simulink model "VSI"  (Simulink 7.6)
settings: Solver=ode23tb  StartTime=0  StopTime=10  MaxStep=5e-6  RelTol=1e-4  AbsTol=1e-5
InitFcn:
  | clear all
  | VSI_AFE_parameters_G1_s
values from neighbouring files (symbols this model uses):
  Cdc_afe = 98.8e-6    (= 9.88e-05)    [VSI_AFE_parameters_G1_s.m]
  DeadTime = 0.0e-6    (= 0)    [VSI_AFE_parameters_G1_s.m]
  f = 400    [VSI_AFE_parameters_G1_s.m]
  La = 1000e-6    (= 0.001)    [VSI_AFE_parameters_G1_s.m]
  Lb = 1000e-6    (= 0.001)    [VSI_AFE_parameters_G1_s.m]
  Lboost_a = 474e-6    (= 0.000474)    [VSI_AFE_parameters_G1_s.m]
  Lboost_b = 471e-6    (= 0.000471)    [VSI_AFE_parameters_G1_s.m]
  Lboost_c = 463e-6    (= 0.000463)    [VSI_AFE_parameters_G1_s.m]
  Lc = 1000e-6    (= 0.001)    [VSI_AFE_parameters_G1_s.m]
  LCdc_afe = 0.65e-6    (= 6.5e-07)    [VSI_AFE_parameters_G1_s.m]
  PWM_Cycle = 4000    [VSI_AFE_parameters_G1_s.m]
  RCdc_afe = 0.049    [VSI_AFE_parameters_G1_s.m]
  Rdc = 96    [VSI_AFE_parameters_G1_s.m]
  RLa = 0.100    (= 0.1)    [VSI_AFE_parameters_G1_s.m]
  RLb = 0.100    (= 0.1)    [VSI_AFE_parameters_G1_s.m]
  RLboost_a = 0.080    (= 0.08)    [VSI_AFE_parameters_G1_s.m]
  RLboost_b = 0.084    [VSI_AFE_parameters_G1_s.m]
  RLboost_c = 0.110    (= 0.11)    [VSI_AFE_parameters_G1_s.m]
  RLc = 0.100    (= 0.1)    [VSI_AFE_parameters_G1_s.m]
  Vdc = 270/1    (= 270)    [VSI_AFE_parameters_G1_s.m]
  Vfd = 0.75    [VSI_AFE_parameters_G1_s.m]
  Vfs = 1.0    (= 1)    [VSI_AFE_parameters_G1_s.m]
  Vsm = Vse*sqrt(2)-8.2/sqrt(2)*Rss    [VSI_AFE_parameters_G1_s.m]
undefined symbols (not defined in the file or in its folder): Cdc, Ldc
libraries: powerlib x55, cstblocks x10, simulink x4, powerlib_extras x1
settings Model: Creator=marko  LastModifiedBy=wenbo
settings SolverCC: MaxConsecutiveMinStep=10  ZeroCrossAlgorithm=Adaptive  AlgebraicLoopSolver=LineSearch
settings DataIOCC: LimitDataPoints=off  SaveOutput=off  SaveTime=off
settings DebuggingCC: IgnoredZcDiagnostic=none  StrictBusMsg=Warning

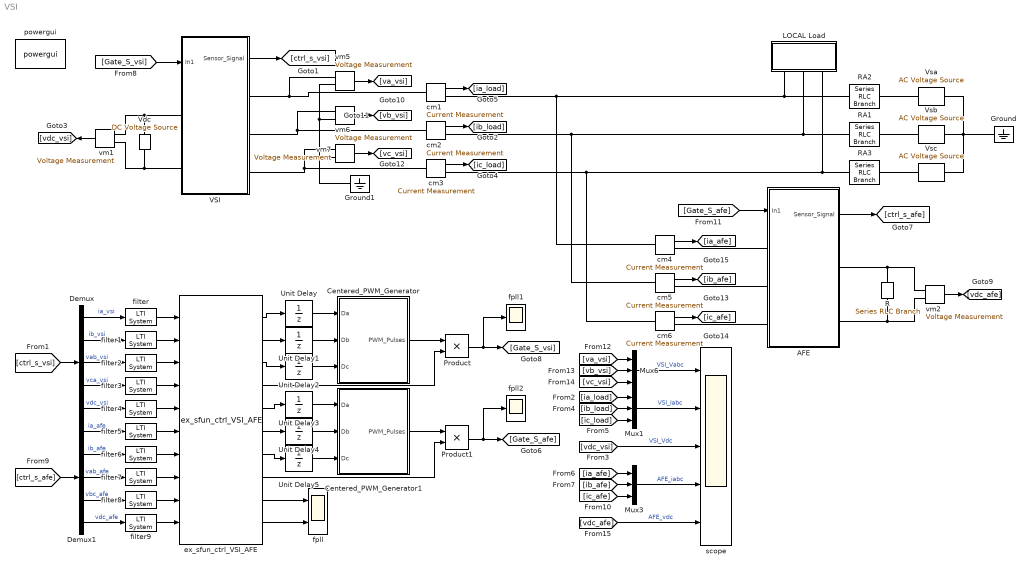
== system VSI ==
  AFE : Subsystem
  Centered_PWM_Generator : Subsystem
  Centered_PWM_Generator1 : Subsystem
  Demux : Demux  Outputs=5
  Demux1 : Demux  Outputs=5
  Ground : powerlib/Elements/Ground  DialogController=POWERSYS.PowerSysDialog  PhysicalDomain=powersysdomain  SubClassName=unknown  LeftPortType=p1  RightPortType=p1  LConnTagsString=a
  Ground1 : powerlib/Elements/Ground  DialogController=POWERSYS.PowerSysDialog  PhysicalDomain=powersysdomain  SubClassName=unknown  LeftPortType=p1  RightPortType=p1  LConnTagsString=a
  LOCAL Load : Subsystem
  Mux1 : Mux  Inputs=3
  Mux3 : Mux  Inputs=3
  Mux6 : Mux  Inputs=3
  Product : Product  RndMeth=Zero
  Product1 : Product  RndMeth=Zero
  R : powerlib/Elements/Series RLC Branch  DialogController=POWERSYS.PowerSysDialog  PhysicalDomain=powersysdomain  SubClassName=unknown  LeftPortType=p1  RightPortType=p1  LConnTagsString=__new0  RConnTagsString=__new0  BranchType=R  Resistance=Rdc  Inductance=Ldc  SetiL0=off  InitialCurrent=0  Capacitance=Cdc  Setx0=off  InitialVoltage=0  Measurements=None
  RA1 : powerlib/Elements/Series RLC Branch  DialogController=POWERSYS.PowerSysDialog  PhysicalDomain=powersysdomain  SubClassName=unknown  LeftPortType=p1  RightPortType=p1  LConnTagsString=__new0  RConnTagsString=__new0  BranchType=R  Resistance=10  Inductance=1e-3  SetiL0=off  InitialCurrent=0  Capacitance=1e-6  Setx0=off  InitialVoltage=0  Measurements=None
  RA2 : powerlib/Elements/Series RLC Branch  DialogController=POWERSYS.PowerSysDialog  PhysicalDomain=powersysdomain  SubClassName=unknown  LeftPortType=p1  RightPortType=p1  LConnTagsString=__new0  RConnTagsString=__new0  BranchType=R  Resistance=10  Inductance=1e-3  SetiL0=off  InitialCurrent=0  Capacitance=1e-6  Setx0=off  InitialVoltage=0  Measurements=None
  RA3 : powerlib/Elements/Series RLC Branch  DialogController=POWERSYS.PowerSysDialog  PhysicalDomain=powersysdomain  SubClassName=unknown  LeftPortType=p1  RightPortType=p1  LConnTagsString=__new0  RConnTagsString=__new0  BranchType=R  Resistance=10  Inductance=1e-3  SetiL0=off  InitialCurrent=0  Capacitance=1e-6  Setx0=off  InitialVoltage=0  Measurements=None
  Unit Delay{,1..5} (6 alike) : UnitDelay  SampleTime=-1
  VSI : Subsystem
  Vdc : powerlib/Electrical Sources/DC Voltage Source  DialogController=POWERSYS.PowerSysDialog  SystemSampleTime=-1  Amplitude=Vdc  Measurements=None
  Vsa : powerlib/Electrical Sources/AC Voltage Source  DialogController=POWERSYS.PowerSysDialog  SystemSampleTime=-1  Amplitude=Vsm  Phase=90  Frequency=f  SampleTime=0  Measurements=None
  Vsb : powerlib/Electrical Sources/AC Voltage Source  DialogController=POWERSYS.PowerSysDialog  SystemSampleTime=-1  Amplitude=Vsm  Phase=90-120  Frequency=f  SampleTime=0  Measurements=None
  Vsc : powerlib/Electrical Sources/AC Voltage Source  DialogController=POWERSYS.PowerSysDialog  SystemSampleTime=-1  Amplitude=Vsm  Phase=90+120  Frequency=f  SampleTime=0  Measurements=None
  cm{1..6} (6 alike) : powerlib/Measurements/Current Measurement  DialogController=POWERSYS.PowerSysDialog  SystemSampleTime=-1  PhasorSimulation=off  OutputType=Complex  PSBequivalent=0
  ex_sfun_ctrl_VSI_AFE : S-Function  FunctionName=ex_sfun_ctrl_VSI_AFE  EnableBusSupport=off  mask(Legacy Function){SFunctionSpec=void epwm1_isr(double y1[1], double y2[1], double y3[1], double y4[1], double y5[1], double y6[1], double y7[1], double y8[1], double y9[1], double u1, double u2, double u3, double u4, double u5, double u6, double u7, double u8, double u9, double u10), ShowSpec=off}
      mask prompts: ShowSpec "Display function specification"
      mask help:
      | This block allows you to call the legacy functions specified by the following Legacy Code Tool definition:
      | def.SFunctionName = 'ex_sfun_ctrl_VSI_AFE';
      | def.OutputFcnSpec = 'void epwm1_isr(double y1[1], double y2[1], double y3[1], double y4[1], double y5[1], double y6[1], double y7[1], double y8[1], double y9[1], double u1, double u2, double u3, double u4, double u5, double u6, double u7, double u8, double u9, double u10)';
      | def.HeaderFiles = {'math.h'};
      | def.SourceFiles = {'epwm1_isr.c'};
      | def.SampleTime = 5e-005;
      mask Help: <p>This block was generated automatically by the Legacy Code Tool. For detailed help on this tool, call<a href="matlab:legacy_code('help')"> legacy_code('help')</a>.</p>
      mask CallbackString:
      | |if strcmp(get_param(gcbh, 'ShowSpec'), 'on')
      |   set_param(gcbh, 'MaskDisplay', sprintf('fprintf(''%s'');', get_param(gcbh, 'SFunctionSpec')));
      | else
      |   set_param(gcbh, 'MaskDisplay', sprintf('fprintf(''%s'');', get_param(gcbh, 'FunctionName')));
      | end
      mask Display: fprintf('ex_sfun_ctrl_VSI_AFE');
  filter{,1..9} (10 alike) : cstblocks/LTI System  SystemSampleTime=-1  sys=tf_filter  IC=[]
  fpll : Scope  NumInputPorts=2
      settings: TimeRange=10  YMin=375~373  YMax=378.25~379.5  SaveName=ia_L
  fpll1 : Scope
      settings: TimeRange=1  YMin=358.141  YMax=395.841  SaveName=ia_L1
  fpll2 : Scope
      settings: TimeRange=1  YMin=358.141  YMax=395.841  SaveName=ia_L2
  powergui : powerlib/powergui  Priority=1  SystemSampleTime=-1  SimulationMode=Continuous  SampleTime=50e-6  frequency=60  SPID=on  DisableSnubberDevices=off  DisableRonSwitches=off  DisableVfSwitches=off  SwTol=0  Interpol=off  frequencyindice=0  echomessages=off  HookPort=off  DisplayEquations=off  FunctionMessages=off  EnableUseOfTLC=off  x0status=blocks  RestoreLinks=warning  ResistiveCurrentMeasurement=off  Frange=[0:2:500]  Ylog=off  Xlog=on  ShowGrid=off  save=off  variable=ZData  structure=ia_L  ZoomFFT=on  StartTime=0.1  cycles=1  DisplayStyle=1  fundamental=400  FreqAxis=off  MaxFrequency=100000  frequencyindicesteady=400  RmsSteady=1  display=off  Ts=0  methode=off
  scope : Scope  NumInputPorts=5
      settings: TimeRange=10  YMin=-100~-15~256.5~-15~0  YMax=100~17.5~283.5~25~250  SaveName=va_ia  MaxDataPoints=2000000
  vm{1..2,5..7} (5 alike) : powerlib/Measurements/Voltage Measurement  DialogController=POWERSYS.PowerSysDialog  SystemSampleTime=-1  PhasorSimulation=off  OutputType=Complex  PSBequivalent=0
  wires:
  vm5/1 -> [va_vsi]
  vm6/1 -> [vb_vsi]
  vm7/1 -> [vc_vsi]
  [va_vsi] -> Mux6/1
  [vb_vsi] -> Mux6/2
  [vc_vsi] -> Mux6/3
  Mux6/1 -> scope/1  "VSI_Vabc"
  Unit Delay/1 -> Centered_PWM_Generator/1(Da)
  Unit Delay1/1 -> Centered_PWM_Generator/2(Db)
  Unit Delay2/1 -> Centered_PWM_Generator/3(Dc)
  Demux/1 -> filter/1  "ia_vsi"
  Demux/2 -> filter1/1  "ib_vsi"
  Demux/3 -> filter2/1  "vab_vsi"
  Demux/4 -> filter3/1  "vca_vsi"
  Demux/5 -> filter4/1  "vdc_vsi"
  VSI/1(Sensor_Signal) -> [ctrl_s_vsi]
  [ctrl_s_vsi] -> Demux/1
  [Gate_S_vsi] -> VSI/1(In1)
  Demux1/1 -> filter5/1  "ia_afe"
  Demux1/2 -> filter6/1  "ib_afe"
  Demux1/3 -> filter7/1  "vab_afe"
  Demux1/4 -> filter8/1  "vbc_afe"
  Demux1/5 -> filter9/1  "vdc_afe"
  [ctrl_s_afe] -> Demux1/1
  ex_sfun_ctrl_VSI_AFE/1 -> Unit Delay/1
  ex_sfun_ctrl_VSI_AFE/2 -> Unit Delay1/1
  ex_sfun_ctrl_VSI_AFE/3 -> Unit Delay2/1
  filter/1 -> ex_sfun_ctrl_VSI_AFE/1
  filter1/1 -> ex_sfun_ctrl_VSI_AFE/2
  filter2/1 -> ex_sfun_ctrl_VSI_AFE/3
  filter3/1 -> ex_sfun_ctrl_VSI_AFE/4
  filter4/1 -> ex_sfun_ctrl_VSI_AFE/5
  filter5/1 -> ex_sfun_ctrl_VSI_AFE/6
  filter6/1 -> ex_sfun_ctrl_VSI_AFE/7
  filter7/1 -> ex_sfun_ctrl_VSI_AFE/8
  filter8/1 -> ex_sfun_ctrl_VSI_AFE/9
  filter9/1 -> ex_sfun_ctrl_VSI_AFE/10
  cm1/1 -> [ia_load]
  [vdc_vsi] -> scope/3  "VSI_Vdc"
  vm1/1 -> [vdc_vsi]
  cm2/1 -> [ib_load]
  cm3/1 -> [ic_load]
  Mux1/1 -> scope/2  "VSI_Iabc"
  [ia_load] -> Mux1/1
  [ib_load] -> Mux1/2
  [ic_load] -> Mux1/3
  Product/1 -> [Gate_S_vsi], fpll1/1
  Centered_PWM_Generator/1(PWM_Pulses) -> Product/1
  ex_sfun_ctrl_VSI_AFE/9 -> fpll/1
  ex_sfun_ctrl_VSI_AFE/10 -> fpll/2
  ex_sfun_ctrl_VSI_AFE/4 -> Product/2
  Unit Delay3/1 -> Centered_PWM_Generator1/1(Da)
  Unit Delay4/1 -> Centered_PWM_Generator1/2(Db)
  Unit Delay5/1 -> Centered_PWM_Generator1/3(Dc)
  Product1/1 -> fpll2/1, [Gate_S_afe]
  Centered_PWM_Generator1/1(PWM_Pulses) -> Product1/1
  ex_sfun_ctrl_VSI_AFE/8 -> Product1/2
  ex_sfun_ctrl_VSI_AFE/5 -> Unit Delay3/1
  ex_sfun_ctrl_VSI_AFE/6 -> Unit Delay4/1
  ex_sfun_ctrl_VSI_AFE/7 -> Unit Delay5/1
  [ia_afe] -> Mux3/1
  [ib_afe] -> Mux3/2
  [ic_afe] -> Mux3/3
  Mux3/1 -> scope/4  "AFE_iabc"
  [vdc_afe] -> scope/5  "AFE_vdc"
  [Gate_S_afe] -> AFE/1(In1)
  AFE/1(Sensor_Signal) -> [ctrl_s_afe]
  vm2/1 -> [vdc_afe]
  cm4/1 -> [ia_afe]
  cm5/1 -> [ib_afe]
  cm6/1 -> [ic_afe]
  connections:
  VSI/LConn1 -- Vdc/RConn1 -- vm1/LConn1
  VSI/LConn2 -- Vdc/LConn1 -- vm1/LConn2
  VSI/RConn3 -- vm7/LConn1 -- cm3/LConn1
  VSI/RConn2 -- vm6/LConn1 -- cm2/LConn1
  cm1/LConn1 -- VSI/RConn1 -- vm5/LConn1
  RA2/RConn1 -- LOCAL Load/LConn1 -- cm1/RConn1 -- cm4/LConn1
  RA1/RConn1 -- LOCAL Load/LConn2 -- cm2/RConn1 -- cm5/LConn1
  RA3/RConn1 -- LOCAL Load/LConn3 -- cm3/RConn1 -- cm6/LConn1
  Vsa/LConn1 -- Vsc/LConn1 -- Vsb/LConn1 -- Ground/LConn1
  vm5/LConn2 -- vm6/LConn2 -- Ground1/LConn1 -- vm7/LConn2
  RA2/LConn1 -- Vsa/RConn1
  Vsb/RConn1 -- RA1/LConn1
  Vsc/RConn1 -- RA3/LConn1
  AFE/RConn2 -- R/RConn1 -- vm2/LConn2
  AFE/RConn1 -- R/LConn1 -- vm2/LConn1
  AFE/LConn1 -- cm4/RConn1
  AFE/LConn2 -- cm5/RConn1
  AFE/LConn3 -- cm6/RConn1

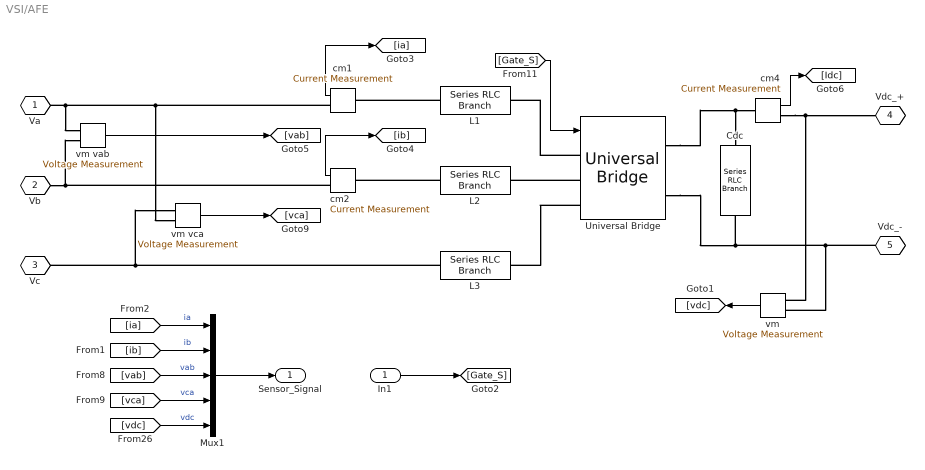
== system VSI/AFE ==
  In1 : Inport
  Cdc : powerlib/Elements/Series RLC Branch  DialogController=POWERSYS.PowerSysDialog  PhysicalDomain=powersysdomain  SubClassName=unknown  LeftPortType=p1  RightPortType=p1  LConnTagsString=__new0  RConnTagsString=__new0  BranchType=C  Resistance=RCdc_afe  Inductance=LCdc_afe  SetiL0=off  InitialCurrent=0  Capacitance=Cdc_afe  Setx0=off  InitialVoltage=0  Measurements=None
  L1 : powerlib/Elements/Series RLC Branch  DialogController=POWERSYS.PowerSysDialog  PhysicalDomain=powersysdomain  SubClassName=unknown  LeftPortType=p1  RightPortType=p1  LConnTagsString=__new0  RConnTagsString=__new0  BranchType=RL  Resistance=RLboost_a  Inductance=Lboost_a  SetiL0=off  InitialCurrent=0  Capacitance=1e-6  Setx0=off  InitialVoltage=0  Measurements=None
  L2 : powerlib/Elements/Series RLC Branch  DialogController=POWERSYS.PowerSysDialog  PhysicalDomain=powersysdomain  SubClassName=unknown  LeftPortType=p1  RightPortType=p1  LConnTagsString=__new0  RConnTagsString=__new0  BranchType=RL  Resistance=RLboost_b  Inductance=Lboost_b  SetiL0=off  InitialCurrent=0  Capacitance=1e-6  Setx0=off  InitialVoltage=0  Measurements=None
  L3 : powerlib/Elements/Series RLC Branch  DialogController=POWERSYS.PowerSysDialog  PhysicalDomain=powersysdomain  SubClassName=unknown  LeftPortType=p1  RightPortType=p1  LConnTagsString=__new0  RConnTagsString=__new0  BranchType=RL  Resistance=RLboost_c  Inductance=Lboost_c  SetiL0=off  InitialCurrent=0  Capacitance=1e-6  Setx0=off  InitialVoltage=0  Measurements=None
  Mux1 : Mux  Inputs=5
  Universal Bridge : powerlib/Power Electronics/Universal Bridge  DialogController=POWERSYS.PowerSysDialog  SystemSampleTime=-1  Arms=3  SnubberResistance=inf  SnubberCapacitance=inf  Device=IGBT / Diodes  Ron=Rsd  Lon=0  ForwardVoltages=[Vfs Vfd]  ForwardVoltage=0  GTOparameters=[ 10e-6 , 20e-6 ]  IGBTparameters=[ 0, 0 ]  Measurements=None  Measurements_2=None  converterType=Rectifier
  cm1 : powerlib/Measurements/Current Measurement  DialogController=POWERSYS.PowerSysDialog  SystemSampleTime=-1  PhasorSimulation=off  OutputType=Complex  PSBequivalent=0
  cm2 : powerlib/Measurements/Current Measurement  DialogController=POWERSYS.PowerSysDialog  SystemSampleTime=-1  PhasorSimulation=off  OutputType=Complex  PSBequivalent=0
  cm4 : powerlib/Measurements/Current Measurement  DialogController=POWERSYS.PowerSysDialog  SystemSampleTime=-1  PhasorSimulation=off  OutputType=Complex  PSBequivalent=0
  vm : powerlib/Measurements/Voltage Measurement  DialogController=POWERSYS.PowerSysDialog  SystemSampleTime=-1  PhasorSimulation=off  OutputType=Complex  PSBequivalent=0
  vm vab : powerlib/Measurements/Voltage Measurement  DialogController=POWERSYS.PowerSysDialog  SystemSampleTime=-1  PhasorSimulation=off  OutputType=Complex  PSBequivalent=0
  vm vca : powerlib/Measurements/Voltage Measurement  DialogController=POWERSYS.PowerSysDialog  SystemSampleTime=-1  PhasorSimulation=off  OutputType=Complex  PSBequivalent=0
  Va : PMIOPort  Tag=PMCPort  Port=1  Side=Left
  Vb : PMIOPort  Tag=PMCPort  Port=2  Side=Left
  Vc : PMIOPort  Tag=PMCPort  Port=3  Side=Left
  Vdc_+ : PMIOPort  Tag=PMCPort  Port=4  Side=Right
  Vdc_- : PMIOPort  Tag=PMCPort  Port=5  Side=Right
  Sensor_Signal : Outport
  wires:
  [Gate_S] -> Universal Bridge/1
  cm4/1 -> [Idc]
  cm1/1 -> [ia]
  cm2/1 -> [ib]
  vm vab/1 -> [vab]
  vm vca/1 -> [vca]
  vm/1 -> [vdc]
  [ia] -> Mux1/1  "ia"
  [ib] -> Mux1/2  "ib"
  [vab] -> Mux1/3  "vab"
  [vca] -> Mux1/4  "vca"
  [vdc] -> Mux1/5  "vdc"
  Mux1/1 -> Sensor_Signal/1
  In1/1 -> [Gate_S]
  connections:
  Universal Bridge/LConn1 -- L1/RConn1
  Universal Bridge/LConn2 -- L2/RConn1
  Universal Bridge/LConn3 -- L3/RConn1
  vm vab/LConn1 -- cm1/RConn1 -- vm vca/LConn2 -- Va/RConn1
  cm2/RConn1 -- Vb/RConn1 -- vm vab/LConn2
  cm4/RConn1 -- Vdc_+/RConn1 -- vm/LConn1
  Vdc_-/RConn1 -- Universal Bridge/RConn2 -- Cdc/RConn1 -- vm/LConn2
  L1/LConn1 -- cm1/LConn1
  L2/LConn1 -- cm2/LConn1
  L3/LConn1 -- Vc/RConn1 -- vm vca/LConn1
  Universal Bridge/RConn1 -- cm4/LConn1 -- Cdc/LConn1

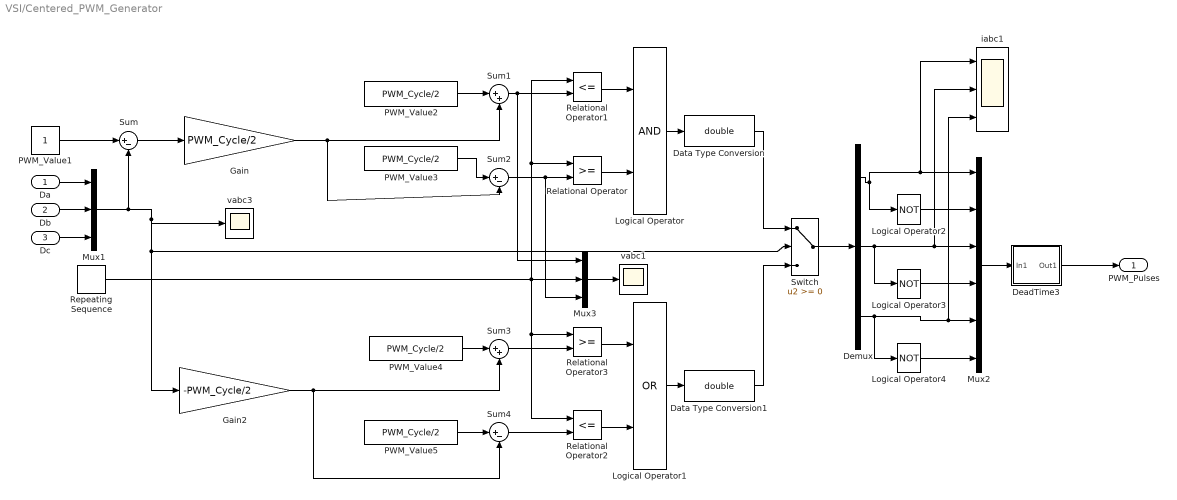
== system VSI/Centered_PWM_Generator ==
  Da : Inport
  Db : Inport  Port=2
  Dc : Inport  Port=3
  Data Type Conversion : DataTypeConversion  OutDataTypeStr=double
  Data Type Conversion1 : DataTypeConversion  OutDataTypeStr=double
  DeadTime3 : Subsystem
  Demux : Demux  Outputs=3
  Gain : Gain  Gain=PWM_Cycle/2
  Gain2 : Gain  Gain=-PWM_Cycle/2
  Logical Operator : Logic  AllPortsSameDT=off  OutDataTypeStr=boolean
  Logical Operator1 : Logic  Operator=OR  AllPortsSameDT=off  OutDataTypeStr=boolean
  Logical Operator2 : Logic  Operator=NOT  OutDataTypeStr=float('double')
  Logical Operator3 : Logic  Operator=NOT  OutDataTypeStr=float('double')
  Logical Operator4 : Logic  Operator=NOT  OutDataTypeStr=float('double')
  Mux1 : Mux  Inputs=3
  Mux2 : Mux  Inputs=6
  Mux3 : Mux  Inputs=3
  PWM_Value1 : Constant
  PWM_Value{2..5} (4 alike) : Constant  Value=PWM_Cycle/2
  Relational Operator : RelationalOperator  OutDataTypeStr=boolean
  Relational Operator1 : RelationalOperator  Operator=<=  OutDataTypeStr=boolean
  Relational Operator2 : RelationalOperator  Operator=<=  OutDataTypeStr=boolean
  Relational Operator3 : RelationalOperator  OutDataTypeStr=boolean
  Repeating Sequence : simulink/Sources/Repeating Sequence  rep_seq_t="[0  (0.5*PWM_Cycle*12.5e-9) (1*PWM_Cycle*12.5e-9)]"  rep_seq_y=[0 PWM_Cycle 0]
  Sum : Sum  Inputs=|+-
  Sum1 : Sum  Inputs=|++
  Sum2 : Sum  Inputs=|+-
  Sum3 : Sum  Inputs=|++
  Sum4 : Sum  Inputs=|+-
  Switch : Switch
  iabc1 : Scope  NumInputPorts=3
      settings: TimeRange=0.02  YMin=-9~-5~-5  YMax=8~5~5  SaveName=iabc_L2
  vabc1 : Scope
      settings: TimeRange=0.01  YMin=0  YMax=4000  SaveName=vabcll2
  vabc3 : Scope
      settings: TimeRange=0.01  YMin=-11  YMax=12  SaveName=vabcll1
  PWM_Pulses : Outport
  wires:
  Logical Operator4/1 -> Mux2/6
  Demux/3 -> Logical Operator4/1, Mux2/5, iabc1/3
  Logical Operator3/1 -> Mux2/4
  Demux/2 -> Logical Operator3/1, Mux2/3, iabc1/2
  Logical Operator2/1 -> Mux2/2
  Demux/1 -> Logical Operator2/1, Mux2/1, iabc1/1
  Mux2/1 -> DeadTime3/1(In1)
  Dc/1 -> Mux1/3
  Db/1 -> Mux1/2
  Da/1 -> Mux1/1
  Mux1/1 -> Sum/2, Switch/2, Gain2/1, vabc3/1
  Switch/1 -> Demux/1
  Data Type Conversion1/1 -> Switch/3
  Gain2/1 -> Sum3/2, Sum4/2
  Logical Operator1/1 -> Data Type Conversion1/1
  Relational Operator2/1 -> Logical Operator1/2
  Relational Operator3/1 -> Logical Operator1/1
  Sum3/1 -> Relational Operator3/2
  Sum4/1 -> Relational Operator2/2
  PWM_Value5/1 -> Sum4/1
  PWM_Value4/1 -> Sum3/1
  Data Type Conversion/1 -> Switch/1
  Logical Operator/1 -> Data Type Conversion/1
  Relational Operator/1 -> Logical Operator/2
  Relational Operator1/1 -> Logical Operator/1
  Sum1/1 -> Relational Operator1/2, Mux3/1
  Sum2/1 -> Relational Operator/2, Mux3/3
  PWM_Value3/1 -> Sum2/1
  Gain/1 -> Sum2/2, Sum1/2
  Sum/1 -> Gain/1
  PWM_Value1/1 -> Sum/1
  Repeating Sequence/1 -> Relational Operator1/1, Relational Operator/1, Relational Operator3/1, Relational Operator2/1, Mux3/2
  DeadTime3/1(Out1) -> PWM_Pulses/1
  PWM_Value2/1 -> Sum1/1
  Mux3/1 -> vabc1/1

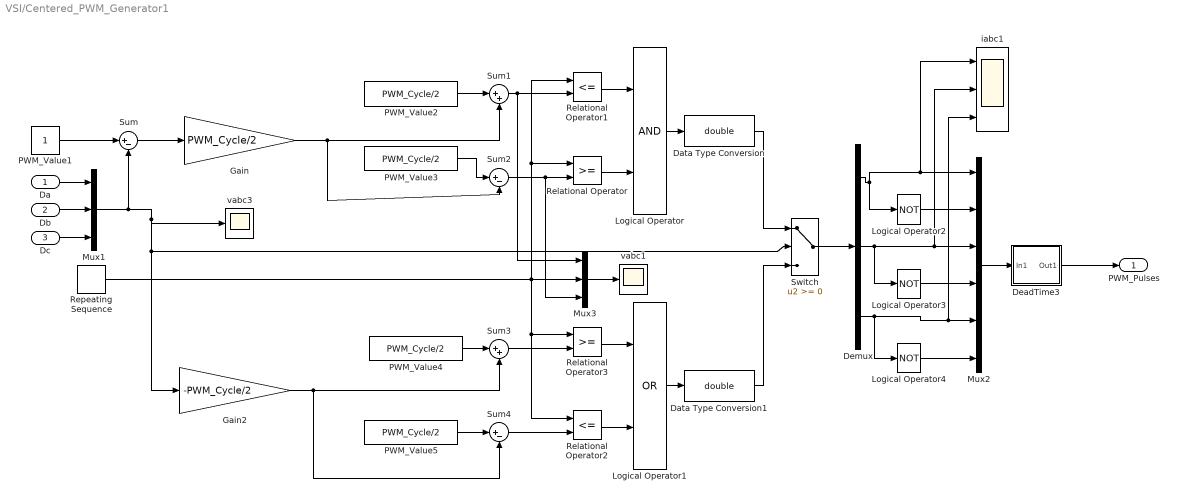
== system VSI/Centered_PWM_Generator1 ==
  Da : Inport
  Db : Inport  Port=2
  Dc : Inport  Port=3
  Data Type Conversion : DataTypeConversion  OutDataTypeStr=double
  Data Type Conversion1 : DataTypeConversion  OutDataTypeStr=double
  DeadTime3 : Subsystem
  Demux : Demux  Outputs=3
  Gain : Gain  Gain=PWM_Cycle/2
  Gain2 : Gain  Gain=-PWM_Cycle/2
  Logical Operator : Logic  AllPortsSameDT=off  OutDataTypeStr=boolean
  Logical Operator1 : Logic  Operator=OR  AllPortsSameDT=off  OutDataTypeStr=boolean
  Logical Operator2 : Logic  Operator=NOT  OutDataTypeStr=float('double')
  Logical Operator3 : Logic  Operator=NOT  OutDataTypeStr=float('double')
  Logical Operator4 : Logic  Operator=NOT  OutDataTypeStr=float('double')
  Mux1 : Mux  Inputs=3
  Mux2 : Mux  Inputs=6
  Mux3 : Mux  Inputs=3
  PWM_Value1 : Constant
  PWM_Value{2..5} (4 alike) : Constant  Value=PWM_Cycle/2
  Relational Operator : RelationalOperator  OutDataTypeStr=boolean
  Relational Operator1 : RelationalOperator  Operator=<=  OutDataTypeStr=boolean
  Relational Operator2 : RelationalOperator  Operator=<=  OutDataTypeStr=boolean
  Relational Operator3 : RelationalOperator  OutDataTypeStr=boolean
  Repeating Sequence : simulink/Sources/Repeating Sequence  rep_seq_t="[0  (0.5*PWM_Cycle*12.5e-9) (1*PWM_Cycle*12.5e-9)]"  rep_seq_y=[0 PWM_Cycle 0]
  Sum : Sum  Inputs=|+-
  Sum1 : Sum  Inputs=|++
  Sum2 : Sum  Inputs=|+-
  Sum3 : Sum  Inputs=|++
  Sum4 : Sum  Inputs=|+-
  Switch : Switch
  iabc1 : Scope  NumInputPorts=3
      settings: TimeRange=0.02  YMin=-9~-5~-5  YMax=8~5~5  SaveName=iabc_L2
  vabc1 : Scope
      settings: TimeRange=0.01  YMin=0  YMax=4000  SaveName=vabcll2
  vabc3 : Scope
      settings: TimeRange=0.01  YMin=-11  YMax=12  SaveName=vabcll1
  PWM_Pulses : Outport
  wires:
  Mux3/1 -> vabc1/1
  PWM_Value2/1 -> Sum1/1
  DeadTime3/1(Out1) -> PWM_Pulses/1
  Repeating Sequence/1 -> Mux3/2, Relational Operator2/1, Relational Operator3/1, Relational Operator/1, Relational Operator1/1
  PWM_Value1/1 -> Sum/1
  Sum/1 -> Gain/1
  Gain/1 -> Sum1/2, Sum2/2
  PWM_Value3/1 -> Sum2/1
  Sum2/1 -> Mux3/3, Relational Operator/2
  Sum1/1 -> Mux3/1, Relational Operator1/2
  Relational Operator1/1 -> Logical Operator/1
  Relational Operator/1 -> Logical Operator/2
  Logical Operator/1 -> Data Type Conversion/1
  Data Type Conversion/1 -> Switch/1
  PWM_Value4/1 -> Sum3/1
  PWM_Value5/1 -> Sum4/1
  Sum4/1 -> Relational Operator2/2
  Sum3/1 -> Relational Operator3/2
  Relational Operator3/1 -> Logical Operator1/1
  Relational Operator2/1 -> Logical Operator1/2
  Logical Operator1/1 -> Data Type Conversion1/1
  Gain2/1 -> Sum4/2, Sum3/2
  Data Type Conversion1/1 -> Switch/3
  Switch/1 -> Demux/1
  Mux1/1 -> vabc3/1, Gain2/1, Switch/2, Sum/2
  Da/1 -> Mux1/1
  Db/1 -> Mux1/2
  Dc/1 -> Mux1/3
  Mux2/1 -> DeadTime3/1(In1)
  Demux/1 -> iabc1/1, Mux2/1, Logical Operator2/1
  Logical Operator2/1 -> Mux2/2
  Demux/2 -> iabc1/2, Mux2/3, Logical Operator3/1
  Logical Operator3/1 -> Mux2/4
  Demux/3 -> iabc1/3, Mux2/5, Logical Operator4/1
  Logical Operator4/1 -> Mux2/6

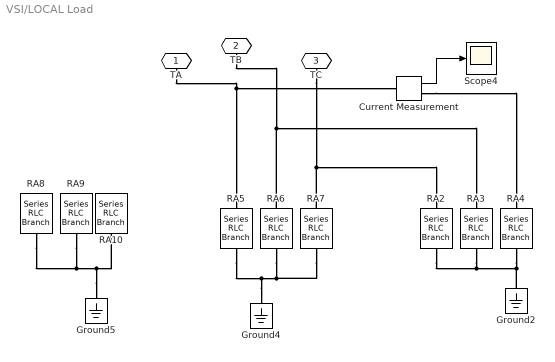
== system VSI/LOCAL Load ==
  Current Measurement : powerlib/Measurements/Current Measurement  DialogController=POWERSYS.PowerSysDialog  SystemSampleTime=-1  PhasorSimulation=off  OutputType=Complex  PSBequivalent=0
  Ground2 : powerlib/Elements/Ground  DialogController=POWERSYS.PowerSysDialog  PhysicalDomain=powersysdomain  SubClassName=unknown  LeftPortType=p1  RightPortType=p1  LConnTagsString=a
  Ground4 : powerlib/Elements/Ground  DialogController=POWERSYS.PowerSysDialog  PhysicalDomain=powersysdomain  SubClassName=unknown  LeftPortType=p1  RightPortType=p1  LConnTagsString=a
  Ground5 : powerlib/Elements/Ground  DialogController=POWERSYS.PowerSysDialog  PhysicalDomain=powersysdomain  SubClassName=unknown  LeftPortType=p1  RightPortType=p1  LConnTagsString=a
  RA10 : powerlib/Elements/Series RLC Branch  DialogController=POWERSYS.PowerSysDialog  PhysicalDomain=powersysdomain  SubClassName=unknown  LeftPortType=p1  RightPortType=p1  LConnTagsString=__new0  RConnTagsString=__new0  BranchType=L  Resistance=0.01e-3  Inductance=80e-3  SetiL0=off  InitialCurrent=0  Capacitance=10e-6  Setx0=off  InitialVoltage=0  Measurements=None
  RA2 : powerlib/Elements/Series RLC Branch  DialogController=POWERSYS.PowerSysDialog  PhysicalDomain=powersysdomain  SubClassName=unknown  LeftPortType=p1  RightPortType=p1  LConnTagsString=__new0  RConnTagsString=__new0  BranchType=R  Resistance=10  Inductance=1e-3  SetiL0=off  InitialCurrent=0  Capacitance=1e-6  Setx0=off  InitialVoltage=0  Measurements=None
  RA3 : powerlib/Elements/Series RLC Branch  DialogController=POWERSYS.PowerSysDialog  PhysicalDomain=powersysdomain  SubClassName=unknown  LeftPortType=p1  RightPortType=p1  LConnTagsString=__new0  RConnTagsString=__new0  BranchType=R  Resistance=10  Inductance=1e-3  SetiL0=off  InitialCurrent=0  Capacitance=1e-6  Setx0=off  InitialVoltage=0  Measurements=None
  RA4 : powerlib/Elements/Series RLC Branch  DialogController=POWERSYS.PowerSysDialog  PhysicalDomain=powersysdomain  SubClassName=unknown  LeftPortType=p1  RightPortType=p1  LConnTagsString=__new0  RConnTagsString=__new0  BranchType=R  Resistance=10  Inductance=1e-3  SetiL0=off  InitialCurrent=0  Capacitance=1e-6  Setx0=off  InitialVoltage=0  Measurements=None
  RA5 : powerlib/Elements/Series RLC Branch  DialogController=POWERSYS.PowerSysDialog  PhysicalDomain=powersysdomain  SubClassName=unknown  LeftPortType=p1  RightPortType=p1  LConnTagsString=__new0  RConnTagsString=__new0  BranchType=C  Resistance=0.01e-3  Inductance=80e-3  SetiL0=off  InitialCurrent=0  Capacitance=50e-6  Setx0=off  InitialVoltage=0  Measurements=None
  RA6 : powerlib/Elements/Series RLC Branch  DialogController=POWERSYS.PowerSysDialog  PhysicalDomain=powersysdomain  SubClassName=unknown  LeftPortType=p1  RightPortType=p1  LConnTagsString=__new0  RConnTagsString=__new0  BranchType=C  Resistance=0.01e-3  Inductance=80e-3  SetiL0=off  InitialCurrent=0  Capacitance=50e-6  Setx0=off  InitialVoltage=0  Measurements=None
  RA7 : powerlib/Elements/Series RLC Branch  DialogController=POWERSYS.PowerSysDialog  PhysicalDomain=powersysdomain  SubClassName=unknown  LeftPortType=p1  RightPortType=p1  LConnTagsString=__new0  RConnTagsString=__new0  BranchType=C  Resistance=0.01e-3  Inductance=80e-3  SetiL0=off  InitialCurrent=0  Capacitance=50e-6  Setx0=off  InitialVoltage=0  Measurements=None
  RA8 : powerlib/Elements/Series RLC Branch  DialogController=POWERSYS.PowerSysDialog  PhysicalDomain=powersysdomain  SubClassName=unknown  LeftPortType=p1  RightPortType=p1  LConnTagsString=__new0  RConnTagsString=__new0  BranchType=L  Resistance=0.01e-3  Inductance=80e-3  SetiL0=off  InitialCurrent=0  Capacitance=10e-6  Setx0=off  InitialVoltage=0  Measurements=None
  RA9 : powerlib/Elements/Series RLC Branch  DialogController=POWERSYS.PowerSysDialog  PhysicalDomain=powersysdomain  SubClassName=unknown  LeftPortType=p1  RightPortType=p1  LConnTagsString=__new0  RConnTagsString=__new0  BranchType=L  Resistance=0.01e-3  Inductance=80e-3  SetiL0=off  InitialCurrent=0  Capacitance=10e-6  Setx0=off  InitialVoltage=0  Measurements=None
  Scope4 : Scope
      settings: TimeRange=0.2371669915529565  YMin=-100  YMax=100  SaveName=ScopeData2
  TA : PMIOPort  Port=1  Side=Left
  TB : PMIOPort  Port=2  Side=Left
  TC : PMIOPort  Port=3  Side=Left
  wires:
  Current Measurement/1 -> Scope4/1
  connections:
  Ground2/LConn1 -- RA2/RConn1 -- RA3/RConn1 -- RA4/RConn1
  Ground4/LConn1 -- RA5/RConn1 -- RA6/RConn1 -- RA7/RConn1
  Ground5/LConn1 -- RA8/RConn1 -- RA9/RConn1 -- RA10/RConn1
  TA/RConn1 -- RA5/LConn1 -- Current Measurement/LConn1
  RA6/LConn1 -- TB/RConn1 -- RA3/LConn1
  RA7/LConn1 -- TC/RConn1 -- RA2/LConn1
  Current Measurement/RConn1 -- RA4/LConn1

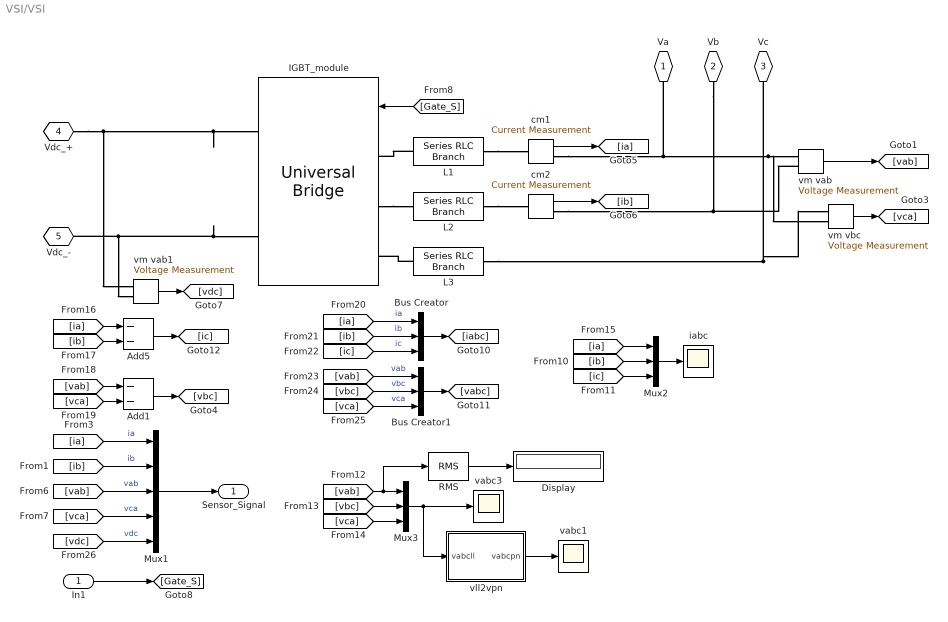
== system VSI/VSI ==
  In1 : Inport
  Add1 : Sum  Inputs=--
  Add5 : Sum  Inputs=--
  Bus Creator : BusCreator  Inputs=3
  Bus Creator1 : BusCreator  Inputs=3
  Display : Display
  IGBT_module : powerlib/Power Electronics/Universal Bridge  DialogController=POWERSYS.PowerSysDialog  SystemSampleTime=-1  Arms=3  SnubberResistance=inf  SnubberCapacitance=inf  Device=IGBT / Diodes  Ron=Rsd  Lon=0  ForwardVoltages=[Vfs Vfd]  ForwardVoltage=0  GTOparameters=[ 10e-6 , 20e-6 ]  IGBTparameters=[ 0, 0 ]  Measurements=None  Measurements_2=None  converterType=Rectifier
  L1 : powerlib/Elements/Series RLC Branch  DialogController=POWERSYS.PowerSysDialog  PhysicalDomain=powersysdomain  SubClassName=unknown  LeftPortType=p1  RightPortType=p1  LConnTagsString=__new0  RConnTagsString=__new0  BranchType=RL  Resistance=RLa  Inductance=La  SetiL0=off  InitialCurrent=0  Capacitance=1e-6  Setx0=off  InitialVoltage=0  Measurements=None
  L2 : powerlib/Elements/Series RLC Branch  DialogController=POWERSYS.PowerSysDialog  PhysicalDomain=powersysdomain  SubClassName=unknown  LeftPortType=p1  RightPortType=p1  LConnTagsString=__new0  RConnTagsString=__new0  BranchType=RL  Resistance=RLb  Inductance=Lb  SetiL0=off  InitialCurrent=0  Capacitance=1e-6  Setx0=off  InitialVoltage=0  Measurements=None
  L3 : powerlib/Elements/Series RLC Branch  DialogController=POWERSYS.PowerSysDialog  PhysicalDomain=powersysdomain  SubClassName=unknown  LeftPortType=p1  RightPortType=p1  LConnTagsString=__new0  RConnTagsString=__new0  BranchType=RL  Resistance=RLc  Inductance=Lc  SetiL0=off  InitialCurrent=0  Capacitance=1e-6  Setx0=off  InitialVoltage=0  Measurements=None
  Mux1 : Mux  Inputs=5
  Mux2 : Mux  Inputs=3
  Mux3 : Mux  Inputs=3
  RMS : powerlib_extras/Measurements/RMS  DialogController=POWERSYS.PowerSysDialog  SystemSampleTime=-1  f1=400
  cm1 : powerlib/Measurements/Current Measurement  DialogController=POWERSYS.PowerSysDialog  SystemSampleTime=-1  PhasorSimulation=off  OutputType=Complex  PSBequivalent=0
  cm2 : powerlib/Measurements/Current Measurement  DialogController=POWERSYS.PowerSysDialog  SystemSampleTime=-1  PhasorSimulation=off  OutputType=Complex  PSBequivalent=0
  iabc : Scope
      settings: TimeRange=0.06  YMin=-10  YMax=10  SaveName=iabc_L
  vabc1 : Scope
      settings: TimeRange=0.01  YMin=-80  YMax=80  SaveName=vabc
  vabc3 : Scope
      settings: TimeRange=0.06  YMin=-300  YMax=225  SaveName=vabcll
  vll2vpn : Subsystem
  vm vab : powerlib/Measurements/Voltage Measurement  DialogController=POWERSYS.PowerSysDialog  SystemSampleTime=-1  PhasorSimulation=off  OutputType=Complex  PSBequivalent=0
  vm vab1 : powerlib/Measurements/Voltage Measurement  DialogController=POWERSYS.PowerSysDialog  SystemSampleTime=-1  PhasorSimulation=off  OutputType=Complex  PSBequivalent=0
  vm vbc : powerlib/Measurements/Voltage Measurement  DialogController=POWERSYS.PowerSysDialog  SystemSampleTime=-1  PhasorSimulation=off  OutputType=Complex  PSBequivalent=0
  Va : PMIOPort  Tag=PMCPort  Port=1  Side=Right
  Vb : PMIOPort  Tag=PMCPort  Port=2  Side=Right
  Vc : PMIOPort  Tag=PMCPort  Port=3  Side=Right
  Vdc_+ : PMIOPort  Tag=PMCPort  Port=4  Side=Left
  Vdc_- : PMIOPort  Tag=PMCPort  Port=5  Side=Left
  Sensor_Signal : Outport
  wires:
  cm1/1 -> [ia]
  [Gate_S] -> IGBT_module/1
  Mux2/1 -> iabc/1
  Mux3/1 -> vabc3/1, vll2vpn/1(vabcll)
  [ia] -> Mux2/1
  [ib] -> Mux2/2
  [ic] -> Mux2/3
  [vab] -> Mux3/1, RMS/1
  [vbc] -> Mux3/2
  [vca] -> Mux3/3
  [ia] -> Bus Creator/1  "ia"
  [ib] -> Bus Creator/2  "ib"
  [ic] -> Bus Creator/3  "ic"
  Bus Creator/1 -> [iabc]
  [vab] -> Bus Creator1/1  "vab"
  [vbc] -> Bus Creator1/2  "vbc"
  [vca] -> Bus Creator1/3  "vca"
  Bus Creator1/1 -> [vabc]
  vll2vpn/1(vabcpn) -> vabc1/1
  RMS/1 -> Display/1
  cm2/1 -> [ib]
  vm vab/1 -> [vab]
  vm vbc/1 -> [vca]
  vm vab1/1 -> [vdc]
  [ia] -> Mux1/1  "ia"
  [ib] -> Mux1/2  "ib"
  [vab] -> Mux1/3  "vab"
  [vca] -> Mux1/4  "vca"
  [vdc] -> Mux1/5  "vdc"
  Mux1/1 -> Sensor_Signal/1
  In1/1 -> [Gate_S]
  Add5/1 -> [ic]
  [ia] -> Add5/1
  [ib] -> Add5/2
  Add1/1 -> [vbc]
  [vab] -> Add1/1
  [vca] -> Add1/2
  connections:
  Va/RConn1 -- cm1/RConn1 -- vm vab/LConn1 -- vm vbc/LConn2
  vm vab/LConn2 -- Vb/RConn1 -- cm2/RConn1
  L1/LConn1 -- IGBT_module/LConn1
  L1/RConn1 -- cm1/LConn1
  L2/RConn1 -- cm2/LConn1
  IGBT_module/LConn2 -- L2/LConn1
  L3/LConn1 -- IGBT_module/LConn3
  Vdc_+/RConn1 -- IGBT_module/RConn1 -- vm vab1/LConn1
  IGBT_module/RConn2 -- Vdc_-/RConn1 -- vm vab1/LConn2
  Vc/RConn1 -- vm vbc/LConn1 -- L3/RConn1

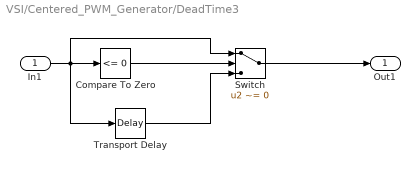
== system VSI/Centered_PWM_Generator/DeadTime3 ==
  In1 : Inport
  Compare To Zero : simulink/Logic and Bit Operations/Compare To Zero  relop=<=  OutDataTypeStr=uint8
  Switch : Switch  Criteria=u2 ~= 0
  Transport Delay : TransportDelay  DelayTime=DeadTime  BufferSize=2048*16  FixedBuffer=on
  Out1 : Outport
  wires:
  Switch/1 -> Out1/1
  Compare To Zero/1 -> Switch/2
  Transport Delay/1 -> Switch/3
  In1/1 -> Transport Delay/1, Compare To Zero/1, Switch/1

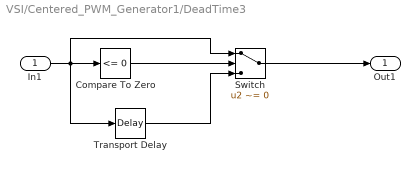
== system VSI/Centered_PWM_Generator1/DeadTime3 ==
  In1 : Inport
  Compare To Zero : simulink/Logic and Bit Operations/Compare To Zero  relop=<=  OutDataTypeStr=uint8
  Switch : Switch  Criteria=u2 ~= 0
  Transport Delay : TransportDelay  DelayTime=DeadTime  BufferSize=2048*16  FixedBuffer=on
  Out1 : Outport
  wires:
  In1/1 -> Switch/1, Compare To Zero/1, Transport Delay/1
  Transport Delay/1 -> Switch/3
  Compare To Zero/1 -> Switch/2
  Switch/1 -> Out1/1

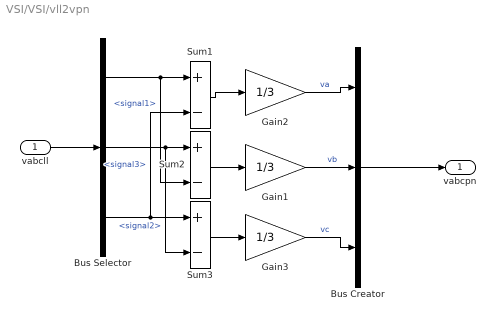
== system VSI/VSI/vll2vpn ==
  vabcll : Inport
  Bus Creator : BusCreator  Inputs=3
  Bus Selector : BusSelector  OutputSignals=signal1,signal2,signal3
  Gain1 : Gain  Gain=1/3
  Gain2 : Gain  Gain=1/3
  Gain3 : Gain  Gain=1/3
  Sum1 : Sum  Inputs=+-
  Sum2 : Sum  Inputs=+-
  Sum3 : Sum  Inputs=+-
  vabcpn : Outport
  wires:
  Bus Creator/1 -> vabcpn/1
  vabcll/1 -> Bus Selector/1
  Bus Selector/1 -> Sum1/1, Sum2/2  "<signal1>"
  Bus Selector/3 -> Sum1/2, Sum3/1  "<signal3>"
  Sum1/1 -> Gain2/1
  Bus Selector/2 -> Sum2/1, Sum3/2  "<signal2>"
  Sum2/1 -> Gain1/1
  Sum3/1 -> Gain3/1
  Gain2/1 -> Bus Creator/1  "va"
  Gain1/1 -> Bus Creator/2  "vb"
  Gain3/1 -> Bus Creator/3  "vc"
